simulink model "tp1ej2pE"  (R2024a)
settings: Solver=VariableStepAuto  StartTime=0.0  StopTime=10.0  RelTol=1e-3
undefined symbols (not defined in the file): b, J, Ks, Kt, L, R
settings Model: Creator=fab  LastModifiedBy=fab

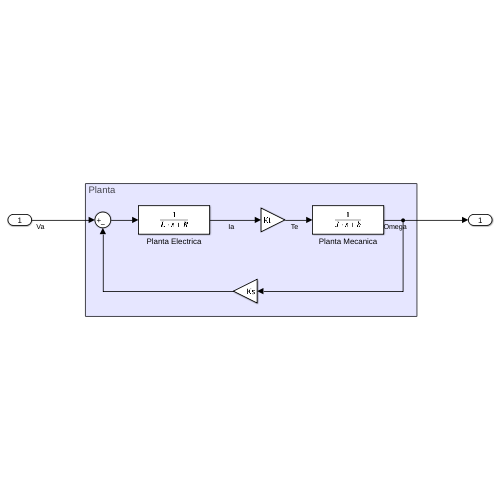
[thumbnail: Simulink's stored preview of the top-level diagram]
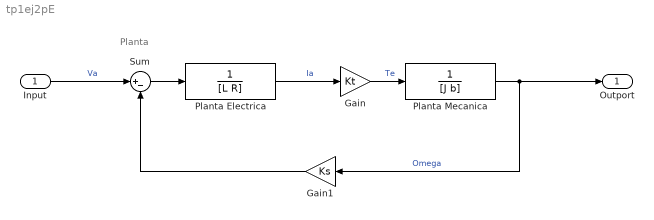
== system tp1ej2pE ==
  note: Planta
  Input : Inport
  Gain : Gain  Gain=Kt
  Gain1 : Gain  Gain=Ks
  Planta Electrica : TransferFcn  Denominator=[L R]
  Planta Mecanica : TransferFcn  Denominator=[J b]
  Sum : Sum  Inputs=|+-
  Outport : Outport
  wires:
  Input/1 -> Sum/1  "Va"
  Planta Mecanica/1 -> Outport/1, Gain1/1  "Omega"
  Planta Electrica/1 -> Gain/1  "Ia"
  Gain1/1 -> Sum/2
  Gain/1 -> Planta Mecanica/1  "Te"
  Sum/1 -> Planta Electrica/1
